simulink model "speed_obs_pll"  (R2023a)
settings: configuration reference "config" (kept outside this file)
model workspace (MAT data in the model file):
  enc_line_inv_p_n = Simulink.Parameter
  enc_line_inv_p_n.Value = 0.0001
  enc_line_inv_p_n.Description = '编码器分辨率 倒数   
    | '
  enc_line_inv_p_n.DataType = 'single'
  enc_line_inv_p_n.Complexity = 'real'
  enc_line_inv_p_n.Dimensions = [1 1]
  init_flag = Simulink.Signal
  init_flag.Description = '初始化信号  0  1 需要被初始化'
  init_flag.DataType = 'uint8'
  init_flag.Dimensions = 1
  init_flag.DimensionsMode = 'auto'
  init_flag.Complexity = 'auto'
  init_flag.SampleTime = -1
  init_flag.SamplingMode = 'auto'
  kFs = Simulink.Parameter
  kFs.Value = 10000
  kFs.Description = '位置环 速度环执行频率  仅用于仿真'
  kFs.DataType = 'double'
  kFs.Complexity = 'real'
  kFs.Dimensions = [1 1]
  tp = Simulink.Parameter
  tp.Value = 0.0001
  tp.Description = '位置环速度环执行周期  s'
  tp.DataType = 'single'
  tp.Complexity = 'real'
  tp.Dimensions = [1 1]
  wn_Hz = Simulink.Parameter
  wn_Hz.Value = 400
  wn_Hz.Description = '速度观测器带宽 Hz'
  wn_Hz.DataType = 'single'
  wn_Hz.Complexity = 'real'
  wn_Hz.Dimensions = [1 1]
libraries: simulink x1
settings Model: DataDictionary=model_config.sldd  ParameterArgumentNames=enc_line_inv_p_n,tp,wn_Hz  Creator=huangcheng  LastModifiedBy=Administrator
settings ConfigSetRef: SourceName=config

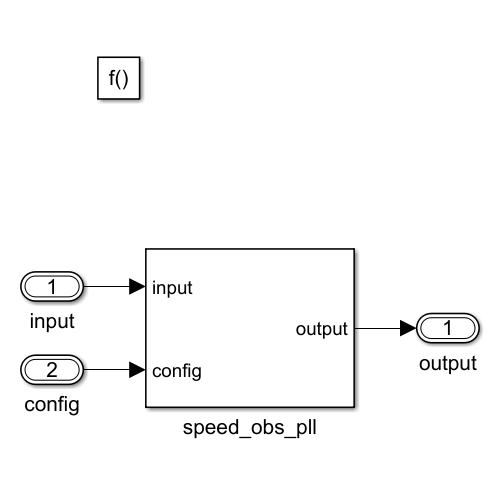
[thumbnail: Simulink's stored preview of the top-level diagram]
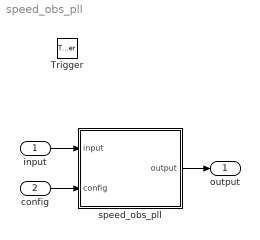
== system speed_obs_pll ==
  input : Inport  OutDataTypeStr=Bus: SpeedObsPllInput  BusOutputAsStruct=on
  config : Inport  Port=2  OutDataTypeStr=Bus: SpeedObsPllConfig  BusOutputAsStruct=on
  Trigger : TriggerPort  TriggerType=function-call  VariantControl=(inherit)  PortDimensions=1
  speed_obs_pll : Subsystem  SystemSampleTime=10e-5
  output : Outport  OutDataTypeStr=Bus: SpeedObsPllOutput  BusOutputAsStruct=on
  wires:
  input/1 -> speed_obs_pll/1(input)
  config/1 -> speed_obs_pll/2(config)
  speed_obs_pll/1(output) -> output/1

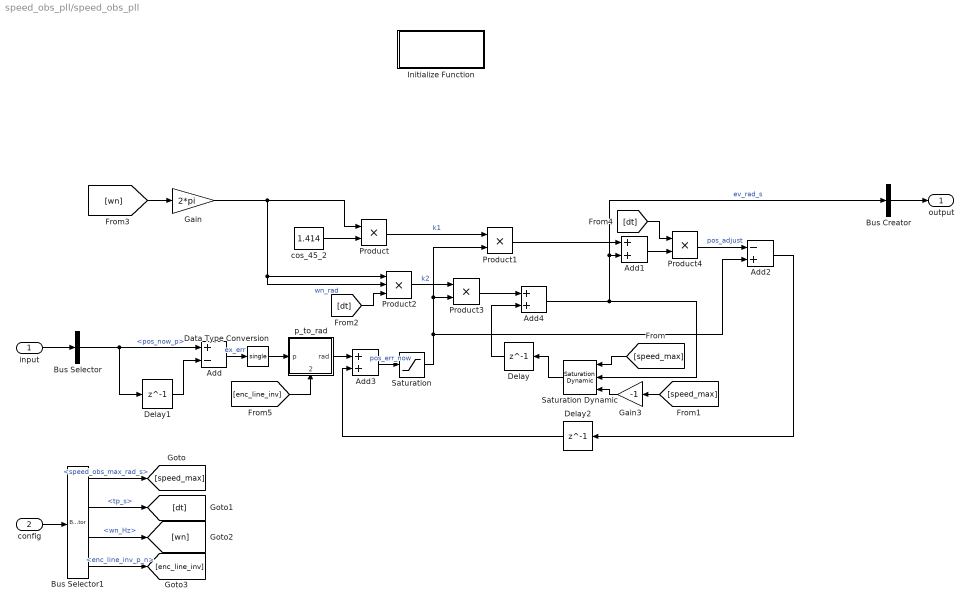
== system speed_obs_pll/speed_obs_pll ==
  input : Inport  OutDataTypeStr=Bus: SpeedObsPllInput  BusOutputAsStruct=on
  config : Inport  Port=2  OutDataTypeStr=Bus: SpeedObsPllConfig  BusOutputAsStruct=on
  Add : Sum  Inputs=+-
  Add1 : Sum
  Add2 : Sum  Inputs=-+
  Add3 : Sum
  Add4 : Sum
  Bus Creator : BusCreator  Inputs=1
  Bus Selector : BusSelector  OutputSignals=pos_now_p
  Bus Selector1 : BusSelector  OutputSignals=speed_obs_max_rad_s,tp_s,wn_Hz,enc_line_inv_p_n
  Data Type Conversion : DataTypeConversion  OutDataTypeStr=single  SaturateOnIntegerOverflow=off  RndMeth=Floor
  Delay : Delay  DelayLength=1  StateName=ev_rad_s_last
  Delay1 : Delay  DelayLength=1  StateName=pos_now_p_last
  Delay2 : Delay  DelayLength=1  StateName=pos_err_last
  Gain : Gain  Gain=2*pi
  Gain3 : Gain  Gain=-1
  Initialize Function : Subsystem  TreatAsAtomicUnit=on
  Product{,1,3..4} (4 alike) : Product
  Product2 : Product  Inputs=3
  Saturation : Saturate  UpperLimit=1  LowerLimit=-1
  Saturation Dynamic : simulink/Discontinuities/Saturation Dynamic  OutMin=[]  OutMax=[]  OutDataTypeStr=Inherit: Same as second input  OutDataType=fixdt(1, 16)  OutScaling=2^-10  DoSatur=off
  cos_45_2 : Constant  Value=1.414  OutDataTypeStr=single
  p_to_rad : Subsystem
      settings: PortSchema="{\"entries\":[{\"content\":{\"sides\":[{\"content\":{\"connectorIds\":[\"In1\"]},\"type\":\"ConnectorPlacement.EquallySpacedRectSide\",\"uuid\":\"452d20cb-539d-4263-99b2-934eba9fec73\"},{\"content\":{\"connectorIds\":[\"Out1\"],\"side\":\"RIGHT\"},\"type\":\"ConnectorPlacement.EquallySpacedRectSide\",\"uuid\":\"b1327dcc-9c06-4e00-8ec6-6c14de84df3d\"},{\"content\":{\"side\":\"TOP\"},\"type\":\"ConnectorPlacement.EquallySpacedRectSide\",\"uuid\":\"c5d938b9-9452-4de9-8cc9-01972dee705b\"},{\"content\":{\"connectorIds\":[\"In2\"],\"side\":\"BOTTOM\"},\"type\":\"ConnectorPlacement.EquallySpacedRectSide\",\"uuid\":\"0f2642f1-d2f6-4884-96ab-f4f81a0f5af5\"}]},\"type\":\"ConnectorPlacement.EquallySpacedConnector\",\"uuid\":\"1c4856e4-e786-4a4d-b510-43c86a79618f\"}],\"packageUris\":[\"http://schema.mathworks.com/mf0/Connector/R2020b\"],\"version\":\"1.0\"}"
  output : Outport  OutDataTypeStr=Bus: SpeedObsPllOutput
  wires:
  cos_45_2/1 -> Product/2
  [wn] -> Gain/1
  Product/1 -> Product1/1  "k1"
  Bus Selector/1 -> Add/1, Delay1/1  "<pos_now_p>"
  Delay1/1 -> Add/2
  Add/1 -> Data Type Conversion/1  "ex_err"
  Data Type Conversion/1 -> p_to_rad/1(p)
  Product2/1 -> Product3/1  "k2"
  Product1/1 -> Add1/1
  Add4/1 -> Saturation Dynamic/2, Bus Creator/1, Add1/2  "ev_rad_s"
  Add1/1 -> Product4/2
  Product4/1 -> Add2/1  "pos_adjust"
  p_to_rad/1(rad) -> Add3/1
  Add3/1 -> Saturation/1  "pos_err_now"
  Delay2/1 -> Add3/2
  Product3/1 -> Add4/1
  Delay/1 -> Add4/2
  Gain/1 -> Product2/1, Product2/2, Product/1  "wn_rad"
  Add2/1 -> Delay2/1
  config/1 -> Bus Selector1/1
  input/1 -> Bus Selector/1
  Bus Selector1/4 -> [enc_line_inv]  "<enc_line_inv_p_n>"
  Bus Selector1/1 -> [speed_max]  "<speed_obs_max_rad_s>"
  Bus Selector1/2 -> [dt]  "<tp_s>"
  Bus Selector1/3 -> [wn]  "<wn_Hz>"
  Bus Creator/1 -> output/1
  Saturation Dynamic/1 -> Delay/1
  [speed_max] -> Saturation Dynamic/1
  [speed_max] -> Gain3/1
  Gain3/1 -> Saturation Dynamic/3
  [dt] -> Product2/3
  [dt] -> Product4/1
  [enc_line_inv] -> p_to_rad/2(enc_line_inv)
  Saturation/1 -> Add2/2, Product3/2, Product1/2

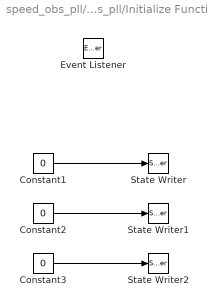
== system speed_obs_pll/speed_obs_pll/Initialize Function ==
  Constant1 : Constant  Value=0  OutDataTypeStr=single
  Constant2 : Constant  Value=0  OutDataTypeStr=int64
  Constant3 : Constant  Value=0  OutDataTypeStr=single
  Event Listener : EventListener  DisableCoverage=on  EventName=reset
  State Writer : StateWriter  StateOwnerBlock=../../Delay  StateName=ev_rad_s_last
  State Writer1 : StateWriter  StateOwnerBlock=../../Delay1  StateName=pos_now_p_last
  State Writer2 : StateWriter  StateOwnerBlock=../../Delay2  StateName=pos_err_last
  wires:
  Constant1/1 -> State Writer/1
  Constant2/1 -> State Writer1/1
  Constant3/1 -> State Writer2/1

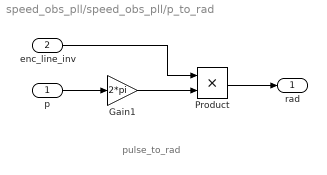
== system speed_obs_pll/speed_obs_pll/p_to_rad ==
  note: pulse_to_rad
  p : Inport
  enc_line_inv : Inport  Port=2
  Gain1 : Gain  Gain=2*pi
  Product : Product
  rad : Outport
  wires:
  p/1 -> Gain1/1
  Gain1/1 -> Product/2
  Product/1 -> rad/1
  enc_line_inv/1 -> Product/1
